simulink model "model_sim"  (R2025b)
settings: Solver=VariableStepAuto  StartTime=0.0  StopTime=10  MaxStep=1e-3  RelTol=1e-3
values from neighbouring files (symbols this model uses):
  balance_deadzone = 1    [simulation__data.m]
  dead_zone_width = double(mod.DEAD_ZONE_WIDTH)    [simulation__data.m]
  dir_coeff = double(mod.direct_conv_fun_coeff)    [simulation__data.m]
  inv_coeff = double(mod.inverse_conv_fun_coeff)    [simulation__data.m]
  Kp = double(mod.Kp)    [simulation__data.m]
  max_PWM = double(mod.MAX_PWM)    [simulation__data.m]
  pulse_zero = pulse_min    (= 10)    [simulation__data.m]
  step_0_pulse_1 = 0    [simulation__data.m]
  step_value = 20    [simulation__data.m]
  x0 = 50    [simulation__data.m]
libraries: simulink x1
settings Model: Creator=feder  LastModifiedBy=Federico Romairone

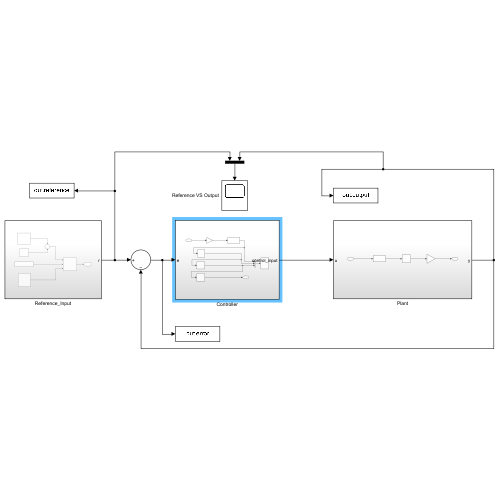
[thumbnail: Simulink's stored preview of the top-level diagram]
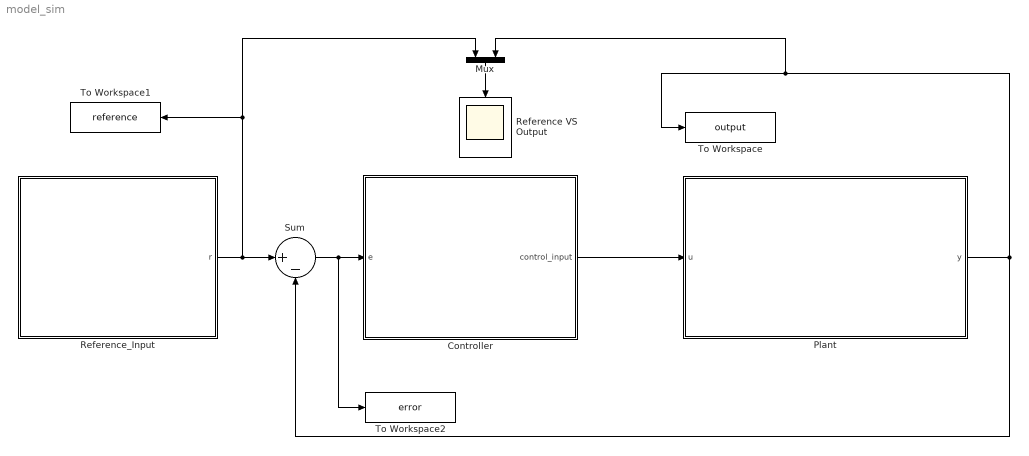
== system model_sim ==
  Controller : Subsystem
  Mux : Mux  Inputs=2
  Plant : Subsystem
  Reference VS Output : Scope
      settings: ActiveDisplayYMinimum=-58.75  ActiveDisplayYMaximum=28.75
  Reference_Input : Subsystem
  Sum : Sum  Inputs=|+-
  To Workspace : ToWorkspace  VariableName=output  SaveFormat=Timeseries  SampleTime=-1
  To Workspace1 : ToWorkspace  VariableName=reference  SaveFormat=Timeseries  SampleTime=-1
  To Workspace2 : ToWorkspace  VariableName=error  SaveFormat=Timeseries  SampleTime=-1
  wires:
  Plant/1(y) -> Mux/2, To Workspace/1, Sum/2
  Sum/1 -> To Workspace2/1, Controller/1(e)
  Controller/1(control_input) -> Plant/1(u)
  Mux/1 -> Reference VS Output/1
  Reference_Input/1(r) -> Mux/1, To Workspace1/1, Sum/1

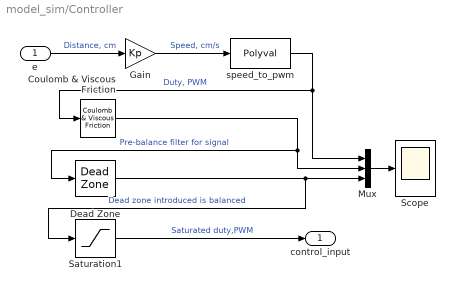
== system model_sim/Controller ==
  e : Inport
  Coulomb & Viscous Friction : simulink/Discontinuities/Coulomb & Viscous Friction  offset=dead_zone_width * balance_deadzone  gain=1
  Dead Zone : DeadZone  LowerValue=-dead_zone_width  UpperValue=dead_zone_width
  Gain : Gain  Gain=Kp
  Mux : Mux  Inputs=3
  Saturation1 : Saturate  UpperLimit=max_PWM  LowerLimit=-max_PWM
  Scope : Scope
      settings: ActiveDisplayYMinimum=-1737.0095805815558  ActiveDisplayYMaximum=6065.0672312742163  DataLoggingVariableName=ScopeData2
  speed_to_pwm : Polyval  Coefs=dir_coeff
  control_input : Outport
  wires:
  e/1 -> Gain/1  "Distance, cm"
  Gain/1 -> speed_to_pwm/1  "Speed, cm/s"
  speed_to_pwm/1 -> Coulomb & Viscous Friction/1, Mux/1  "Duty, PWM"
  Saturation1/1 -> control_input/1  "Saturated duty,PWM"
  Mux/1 -> Scope/1
  Coulomb & Viscous Friction/1 -> Mux/2, Dead Zone/1  "Pre-balance filter for signal"
  Dead Zone/1 -> Mux/3, Saturation1/1  "Dead zone introduced is balanced"

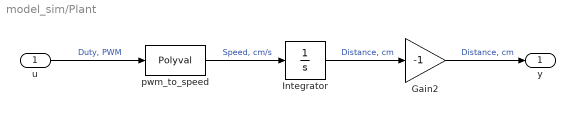
== system model_sim/Plant ==
  u : Inport
  Gain2 : Gain  Gain=-1
  Integrator : Integrator  InitialCondition=-x0
  pwm_to_speed : Polyval  Coefs=inv_coeff
  y : Outport
  wires:
  Integrator/1 -> Gain2/1  "Distance, cm"
  pwm_to_speed/1 -> Integrator/1  "Speed, cm/s"
  Gain2/1 -> y/1  "Distance, cm"
  u/1 -> pwm_to_speed/1  "Duty, PWM"

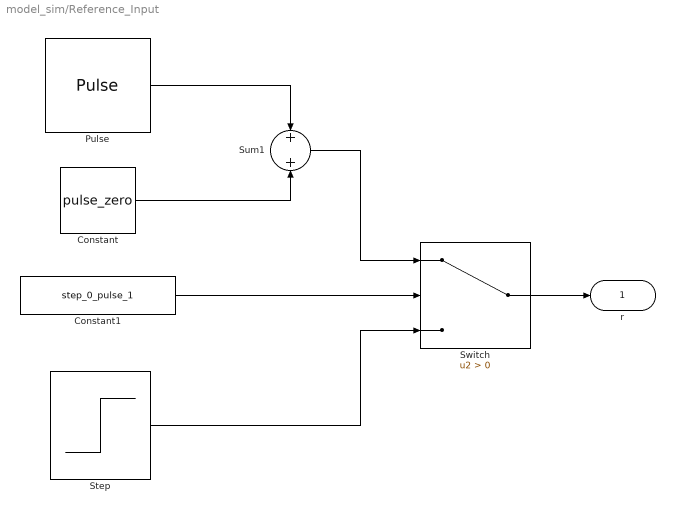
== system model_sim/Reference_Input ==
  Constant : Constant  Value=pulse_zero
  Constant1 : Constant  Value=step_0_pulse_1
  Pulse : DiscretePulseGenerator  PulseType=Time based  Amplitude=step_value  Period=4  PulseWidth=50
  Step : Step  Time=0  After=step_value  SampleTime=0
  Sum1 : Sum
  Switch : Switch  Criteria=u2 > Threshold  SaturateOnIntegerOverflow=off  InputSameDT=off
  r : Outport
  wires:
  Pulse/1 -> Sum1/1
  Constant/1 -> Sum1/2
  Constant1/1 -> Switch/2
  Sum1/1 -> Switch/1
  Step/1 -> Switch/3
  Switch/1 -> r/1
